simulink model "Actuator_model"  (R2015b)
settings: Solver=VariableStepAuto  StartTime=0.0  StopTime=20.0  RelTol=1e-3
values from neighbouring files (symbols this model uses):
  Bv = 10 / ((180/pi) * 1000)    (= 0.000174532925199)    [initialize_param_mdeg.m]    (also in intialize_param.m = 8)
  Jeq = 0.2740    (= 0.274)    [initialize_param_mdeg.m]    (also in intialize_param.m)
  Km = 0.0429    [initialize_param_mdeg.m]    (also in intialize_param.m)
  Kp = wn / (2*zeta)    (= 4297183.46348)    [initialize_param_mdeg.m]    (also in intialize_param.m = 50)
  Kr = 160    [initialize_param_mdeg.m]    (also in intialize_param.m)
  Kv = wn^2 * Bv / (Kp*Kr*Km)    (= 437.062937063)    [initialize_param_mdeg.m]    (also in intialize_param.m = 233.1002331)
  Tv = (Jeq/Bv)    (= 1569.90435866)    [initialize_param_mdeg.m]    (also in intialize_param.m = 0.03425)
undefined symbols (not defined in the file or in its folder): sigbuilder_block
settings Model: Creator=mohit  LastModifiedBy=mohit

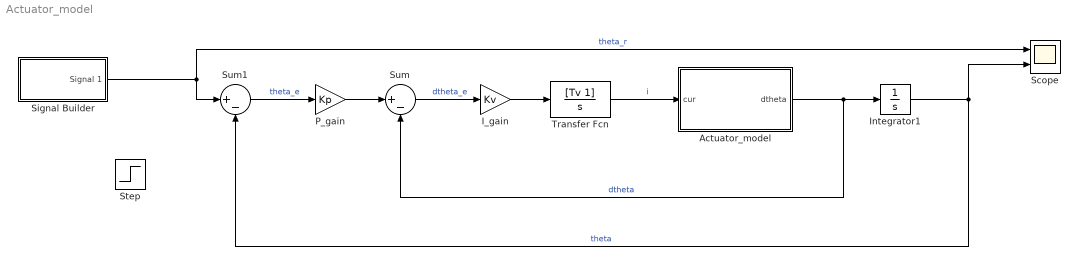
== system Actuator_model ==
  Actuator_model : Subsystem
  I_gain : Gain  Gain=Kv
  Integrator1 : Integrator
  P_gain : Gain  Gain=Kp
  Scope : Scope  NumInputPorts=2
  Signal Builder : Subsystem  Tag=STV Subsys  LoadFcn=sigbuilder_block('load');  StartFcn=sigbuilder_block('start');  StopFcn=sigbuilder_block('stop');  ClipboardFcn=sigbuilder_block('clipboard');  mask(Sigbuilder block){}
      mask help: Simulink:masks:SigbuilderBlock_MD
      mask init:
      | if ~strcmp(get_param(bdroot(gcbh),'SimulationStatus'),'stopped') tuvar = sigbuilder_block('maskInit'); end
      settings: CopyFcn=sigbuilder_block('copy');  DeleteFcn=sigbuilder_block('delete');  ModelCloseFcn=sigbuilder_block('modelClose');  PreSaveFcn=sigbuilder_block('preSave');  PauseFcn=sigbuilder_block('pause');  ContinueFcn=sigbuilder_block('continue');  NameChangeFcn=sigbuilder_block('namechange');  OpenFcn=sigbuilder_block('open',[437.6 199.2 550.4 400 ]);  CloseFcn=sigbuilder_block('close');
      mask Display: plot(0, 0, 100, 100,[2, 2, 32, 32, 2], [68, 8, 8, 68, 68],[32, 2], [38, 38], [32, 19, 2],[53, 60, 44], [32, 17, 17, 2],[16, 16, 31, 31]);txt = getActiveGroup(gcbh);text(2, 100, txt,'verticalAlignment', 'top');
  Step : Step  Time=2  SampleTime=0
  Sum : Sum  Inputs=|+-
  Sum1 : Sum  Inputs=|+-
  Transfer Fcn : TransferFcn  Numerator=[Tv 1]  Denominator=[1 0]
  wires:
  Integrator1/1 -> Scope/2, Sum1/2  "theta"
  Actuator_model/1(dtheta) -> Sum/2, Integrator1/1  "dtheta"
  Transfer Fcn/1 -> Actuator_model/1(cur)  "i"
  Sum/1 -> I_gain/1  "dtheta_e"
  I_gain/1 -> Transfer Fcn/1
  P_gain/1 -> Sum/1
  Sum1/1 -> P_gain/1  "theta_e"
  Signal Builder/1(Signal 1) -> Sum1/1, Scope/1  "theta_r"

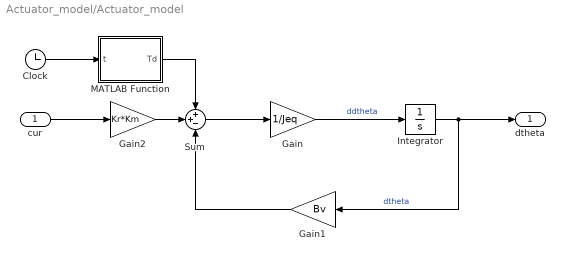
== system Actuator_model/Actuator_model ==
  cur : Inport
  Clock : Clock
  Gain : Gain  Gain=1/Jeq
  Gain1 : Gain  Gain=Bv
  Gain2 : Gain  Gain=Kr*Km
  Integrator : Integrator
  MATLAB Function : MATLAB Function  TreatAsAtomicUnit=on
  Sum : Sum  Inputs=++-
  dtheta : Outport
  wires:
  Gain2/1 -> Sum/2
  Integrator/1 -> dtheta/1, Gain1/1  "dtheta"
  Sum/1 -> Gain/1
  Gain1/1 -> Sum/3
  cur/1 -> Gain2/1
  Gain/1 -> Integrator/1  "ddtheta"
  Clock/1 -> MATLAB Function/1(t)
  MATLAB Function/1(Td) -> Sum/1

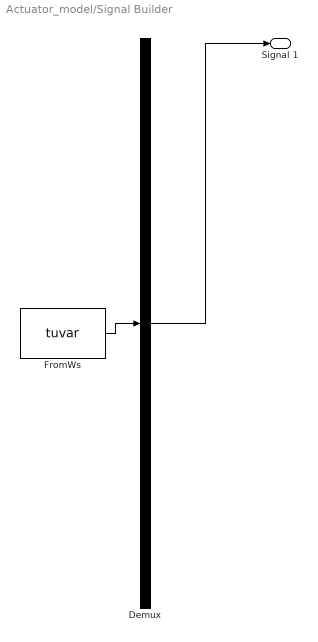
== system Actuator_model/Signal Builder ==
  Demux : Demux  Tag=STV Demux  Outputs=1
  FromWs : FromWorkspace  Tag=STV FromWs  VariableName=tuvar  SampleTime=0
      SigBuilderData=|
      | common.afterFinalStr = 'Extrapolate'
      | common.sampleTime = 0
      | dataSet.timeRange = [0 10]
      | dataSet.name = 'Group 1'
      | sbobj.Groups.Name = 'Group 1'
      | sbobj.Groups.Signals.Name = 'Signal 1'
      | sbobj.Groups.Signals.XData = [0 2 2.05 2.1 2.15 2.2 2.3 2.55 2.65 2.75 2.9 4 4.4 5.05 6 10]
      | sbobj.Groups.Signals.YData = [0 0 0 0.01 0.03 0.09 0.22 0.67 0.88 0.98 1 1 1 1 1 1]
  Signal 1 : Outport  Tag=STV Outport
  wires:
  Demux/1 -> Signal 1/1
  FromWs/1 -> Demux/1

== matlab function Actuator_model/MATLAB Function ==
  data: Td output; t input
function Td = gen_dist(t)
%#codegen

% t = 0:0.004:20
if t > 5 & t < 10
    Td = -1;
else
    Td = 0;
end
end
